simulink model "Sistemaelectro"  (R2023a)
settings: Solver=VariableStepAuto  StartTime=0.0  StopTime=10.0  RelTol=1e-3
values from neighbouring files (symbols this model uses):
  b = 0.0012    [ELEMEC.m]
  J = 0.001    [ELEMEC.m]
  Ke = 0.01    [ELEMEC.m]
  Kt = 0.01    [ELEMEC.m]
  La = 0.023    [ELEMEC.m]
  Ra = 2    [ELEMEC.m]
settings Model: Creator=mluser  LastModifiedBy=fermo

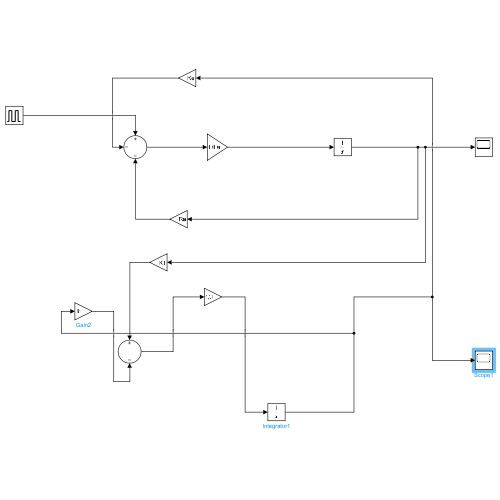
[thumbnail: Simulink's stored preview of the top-level diagram]
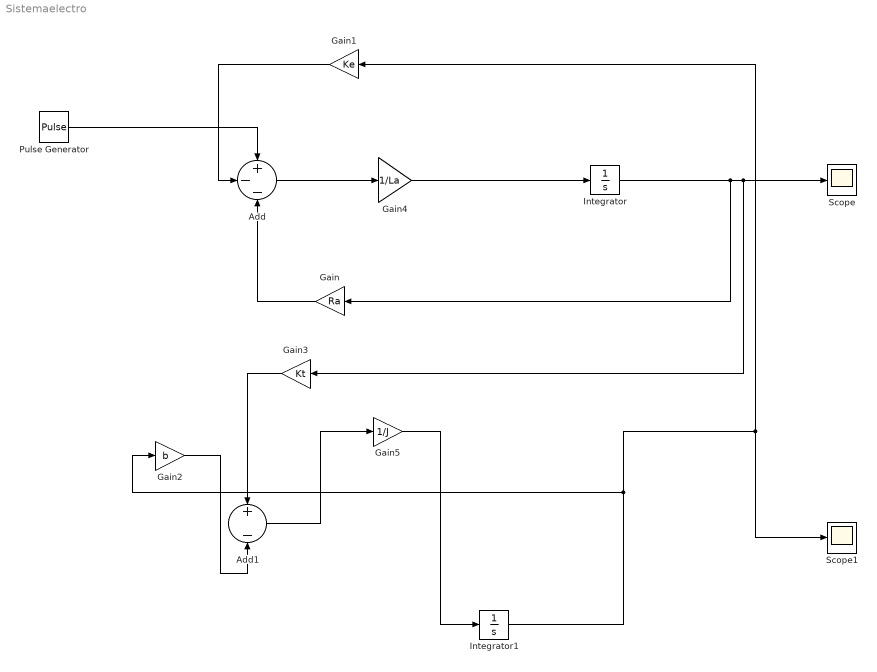
== system Sistemaelectro ==
  Add : Sum  Inputs=+--
  Add1 : Sum  Inputs=+-
  Gain : Gain  Gain=Ra
  Gain1 : Gain  Gain=Ke
  Gain2 : Gain  Gain=b
  Gain3 : Gain  Gain=Kt
  Gain4 : Gain  Gain=1/La
  Gain5 : Gain  Gain=1/J
  Integrator : Integrator
  Integrator1 : Integrator
  Pulse Generator : DiscretePulseGenerator  PulseType=Time based  Amplitude=24  Period=1/20000  PulseWidth=25
  Scope : Scope
  Scope1 : Scope
  wires:
  Add/1 -> Gain4/1
  Gain/1 -> Add/3
  Integrator1/1 -> Gain1/1, Scope1/1, Gain2/1
  Gain1/1 -> Add/2
  Integrator/1 -> Gain/1, Scope/1, Gain3/1
  Add1/1 -> Gain5/1
  Gain2/1 -> Add1/2
  Gain3/1 -> Add1/1
  Gain4/1 -> Integrator/1
  Gain5/1 -> Integrator1/1
  Pulse Generator/1 -> Add/1
